simulink library "AnnSteeringBtc"  (R2022b)
settings: Solver=VariableStepAuto  StartTime=0.0  StopTime=10.0  RelTol=1e-3
undefined symbols (not defined in the file or in its folder): frameSize
libraries: dspindex x2, AudioStats x1, FeaturePath x1, HandyTextFile x1, RTC x1
settings Model: Creator=kl13806  LastModifiedBy=kl13806
settings SolverCC: AlgebraicLoopSolver=TrustRegion
settings DebuggingCC: UnconnectedInputMsg=warning  UnconnectedOutputMsg=warning  UnconnectedLineMsg=warning  SFMachineParentedDataDiag=warning
settings ModelReferenceCC: EnableRefExpFcnMdlSchedulingChecks=on
settings RTWCC: DLArmComputeVersion=19.05

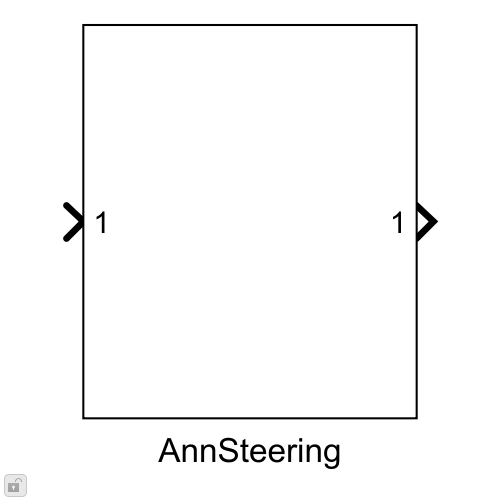
[thumbnail: Simulink's stored preview of the top-level diagram]
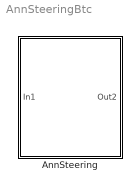
== system AnnSteeringBtc ==
  AnnSteering : Subsystem  mask(Blocklib AnnSteering){Config=[], FeatureName=Steering}
      mask prompts: Config "AnnSteeringConfig"; FeatureName "Feature path name:"
      mask init:
      | blkh=gcbh;
      | Config=BTConfig.Assert(blkh,Config);
      | %Min value to ramp up from
      | minValue = 10^(Config.MinGainDb/20);
      | Config.Validate();
      | BTConfig.InitSetFeatureIfPresent(blkh,'FeatureName');
      mask Callback Config: BTConfig.CallbackHideIfPresent(gcbh,{'FeatureName'});
      mask TypeOptions FeatureName: FeaturePath/FeatureName

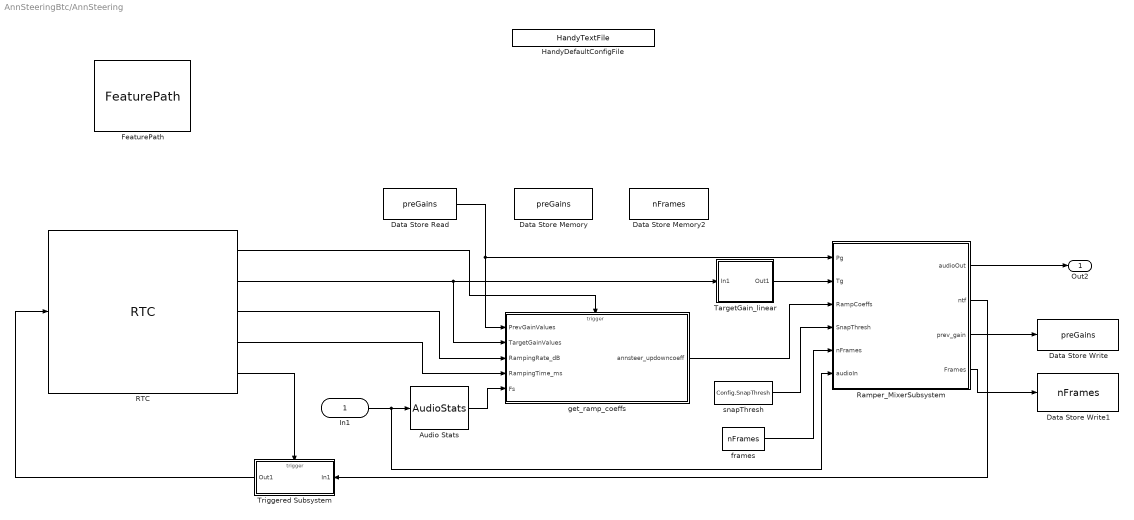
== system AnnSteeringBtc/AnnSteering ==
  In1 : Inport
  Audio Stats : AudioStats/AudioStats  DoSampleRate=on  TypeSampleRate=Inherit: auto  DoCallRate=off  TypeCallRate=Inherit: auto  DoFrameSize=off  TypeFrameSize=Inherit: auto  DoChannelCount=off  TypeChannelCount=Inherit: auto  DoTaskRateFactor=off  TypeTaskRateFactor=Inherit: auto  MacroNameRoot=AUDIO  MacroNameRootEval='AUDIO'  IsMacroNameEval=off  MacroSampleRate=off  MacroCallRate=off  MacroFrameSize=off  MacroChannelCount=off  MacroTaskRateFactor=off  MacroTaskId=off  ValidateSampleRate=off  ValueSampleRate=[]  ValidateCallRate=off  ValueCallRate=[]  ValidateFrameSize=off  ValueFrameSize=[]  ValidateChannelCount=off  ValueChannelCount=[]  ValidateTaskRateFactor=off  ValueTaskRateFactor=[]
  Data Store Memory : DataStoreMemory  DataStoreName=preGains  WriteAfterWriteMsg=warning  InitialValue=Config.Prevgainvalues  ShowAdditionalParam=off  OutDataTypeStr=single
  Data Store Memory2 : DataStoreMemory  DataStoreName=nFrames  InitialValue=zeros(Config.NumAnnOut,Config.NumAnnIn)  ShowAdditionalParam=off  OutDataTypeStr=single
  Data Store Read : DataStoreRead  DataStoreName=preGains  IndexOptions=Index vector (dialog)  Indices=1  OutputSizes=1
  Data Store Write : DataStoreWrite  DataStoreName=preGains  IndexOptions=Index vector (dialog)  Indices=1  OutputSizes=1
  Data Store Write1 : DataStoreWrite  DataStoreName=nFrames  IndexOptions=Index vector (dialog)  Indices=1  OutputSizes=1
  FeaturePath : FeaturePath/FeaturePath  FeatureName=Steering  IsGroup=off  GroupNumber=-1  IsModule=off  TriggerInit=[-245 19 -120 111]
  HandyDefaultConfigFile : HandyTextFile/HandyTextFile  TemplateSource=Config  FileSuffix=Init  OpenDialogOnLoad=off  UseThisBlockName=off  TheDefaultText=|  ShowInLibBrowser=on
      | % $(FILENAME) Setup model parameters for each "Init" callback (e.g. update diagram)
      | sample_rate_in_hertz = 44100;
      | frame_size = 32;
      | sysin_channel_count = 2;
  RTC : RTC/RTC  REQ_Priority=RTC_Mask.NormalPriority  RequestAtInit=off  EnableRequest=on  REQElemName1=target_gain_rtc  REQElemType1=single  REQElemWidth1=length(Config.InitialTargetGainRtc)  REQElemInitial1=Config.InitialTargetGainRtc  REQElemName2=annsteer_rampingRate_rtc  REQElemType2=uint32  REQElemWidth2=length(Config.InitialRampingRateRtc)  REQElemInitial2=Config.InitialRampingRateRtc  REQElemName3=annsteer_rampingTime_rtc  REQElemType3=uint32  REQElemWidth3=length(Config.InitialRampingTimeRtc)  REQElemInitial3=Config.InitialRampingTimeRtc  REQElemType4=uint32  REQElemWidth4=1  REQElemInitial4=[]  REQElemType5=uint32  REQElemWidth5=1  REQElemInitial5=[]  REQElemType6=uint32  REQElemWidth6=1  REQElemInitial6=[]  REQElemType7=uint32  REQElemWidth7=1  REQElemInitial7=[]  REQElemType8=uint32  REQElemWidth8=1  REQElemInitial8=[]  REQElemType9=uint32  REQElemWidth9=1  REQElemInitial9=[]  REQElemType10=uint32  REQElemWidth10=1  REQElemInitial10=[]  EnableResponse=on  EnableRSP_StatusIn=off  RSPElemType1=uint32  RSPElemWidth1=1  RSPElemType2=uint32  RSPElemWidth2=1  RSPElemType3=uint32  RSPElemWidth3=1  RSPElemType4=uint32  RSPElemWidth4=1  RSPElemType5=uint32  RSPElemWidth5=1  RSPElemType6=uint32  RSPElemWidth6=1  RSPElemType7=uint32  RSPElemWidth7=1  RSPElemType8=uint32  RSPElemWidth8=1  RSPElemType9=uint32  RSPElemWidth9=1  RSPElemType10=uint32  RSPElemWidth10=1  EnableNotification=on  EnableNTF_PrepTrig=off  NTFElemType1=uint32  NTFElemWidth1=1  NTFElemType2=uint32  NTFElemWidth2=1  NTFElemType3=uint32  NTFElemWidth3=1  NTFElemType4=uint32  NTFElemWidth4=1  NTFElemType5=uint32  NTFElemWidth5=1  NTFElemType6=uint32  NTFElemWidth6=1  NTFElemType7=uint32  NTFElemWidth7=1  NTFElemType8=uint32  NTFElemWidth8=1  NTFElemType9=uint32  NTFElemWidth9=1  NTFElemType10=uint32  NTFElemWidth10=1  MaskMessageName=Set
  Ramper_MixerSubsystem : Subsystem  TreatAsAtomicUnit=on
  TargetGain_linear : Subsystem
  Triggered Subsystem : Subsystem  TreatAsAtomicUnit=on
  frames : DataStoreRead  DataStoreName=nFrames  IndexOptions=Index vector (dialog)  Indices=1  OutputSizes=1
  get_ramp_coeffs : MATLAB Function  TreatAsAtomicUnit=on
  snapThresh : Constant  Value=Config.SnapThresh  VectorParams1D=off  OutDataTypeStr=single
  Out2 : Outport  VectorParamsAs1DForOutWhenUnconnected=off
  wires:
  RTC/2 -> TargetGain_linear/1(In1), get_ramp_coeffs/2(TargetGainValues)
  Ramper_MixerSubsystem/1(audioOut) -> Out2/1
  Data Store Read/1 -> get_ramp_coeffs/1(PrevGainValues), Ramper_MixerSubsystem/1(Pg)
  RTC/3 -> get_ramp_coeffs/3(RampingRate_dB)
  snapThresh/1 -> Ramper_MixerSubsystem/4(SnapThresh)
  In1/1 -> Ramper_MixerSubsystem/6(audioIn), Audio Stats/1
  Ramper_MixerSubsystem/2(ntf) -> Triggered Subsystem/1(In1)
  RTC/5 -> Triggered Subsystem/Trigger
  Triggered Subsystem/1(Out1) -> RTC/1
  get_ramp_coeffs/1(annsteer_updowncoeff) -> Ramper_MixerSubsystem/3(RampCoeffs)
  Audio Stats/1 -> get_ramp_coeffs/5(Fs)
  Ramper_MixerSubsystem/3(prev_gain) -> Data Store Write/1
  RTC/4 -> get_ramp_coeffs/4(RampingTime_ms)
  RTC/1 -> get_ramp_coeffs/Trigger
  TargetGain_linear/1(Out1) -> Ramper_MixerSubsystem/2(Tg)
  frames/1 -> Ramper_MixerSubsystem/5(nFrames)
  Ramper_MixerSubsystem/4(Frames) -> Data Store Write1/1

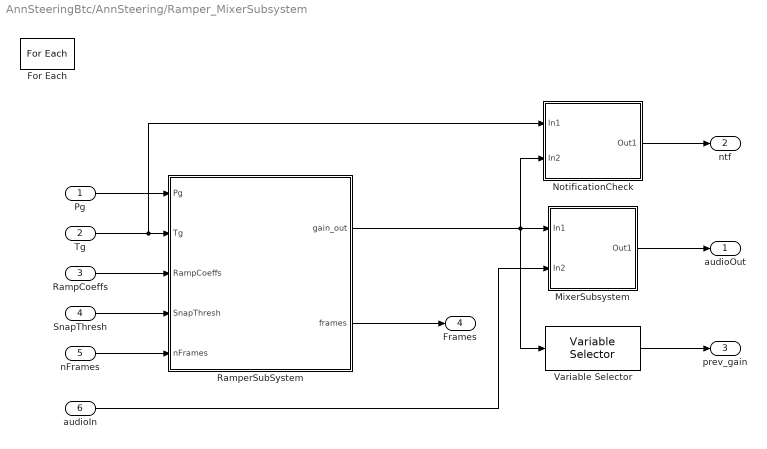
== system AnnSteeringBtc/AnnSteering/Ramper_MixerSubsystem ==
  Pg : Inport  Partition=on  PartitionDimension=1  PartitionWidth=1  PartitionOffset=0
  Tg : Inport  Port=2  Partition=on  PartitionDimension=1  PartitionWidth=1  PartitionOffset=0
  RampCoeffs : Inport  Port=3  Partition=on  PartitionDimension=1  PartitionWidth=1  PartitionOffset=0
  SnapThresh : Inport  Port=4  Partition=on  PartitionDimension=1  PartitionWidth=1  PartitionOffset=0
  nFrames : Inport  Port=5  Partition=on  PartitionDimension=1  PartitionWidth=1  PartitionOffset=0
  audioIn : Inport  Port=6
  For Each : ForEach  DisableCoverage=on
  MixerSubsystem : Subsystem
  NotificationCheck : Subsystem
  RamperSubSystem : Subsystem  TreatAsAtomicUnit=on
  Variable Selector : dspindex/Variable Selector  NumInputs=1  rowsOrCols=Rows  IdxMode=Fixed  Elements=Config.FrameSize  ZerOneIdxMode=One-based  errmode=Clip Index  FillMode=on  FillValues=0
  audioOut : Outport  ConcatenationDimension=2  VectorParamsAs1DForOutWhenUnconnected=off
  ntf : Outport  Port=2  ConcatenationDimension=2  VectorParamsAs1DForOutWhenUnconnected=off
  prev_gain : Outport  Port=3  ConcatenationDimension=1  VectorParamsAs1DForOutWhenUnconnected=off
  Frames : Outport  Port=4  ConcatenationDimension=1  VectorParamsAs1DForOutWhenUnconnected=off
  wires:
  RampCoeffs/1 -> RamperSubSystem/3(RampCoeffs)
  Tg/1 -> RamperSubSystem/2(Tg), NotificationCheck/1(In1)
  Pg/1 -> RamperSubSystem/1(Pg)
  SnapThresh/1 -> RamperSubSystem/4(SnapThresh)
  RamperSubSystem/1(gain_out) -> Variable Selector/1, MixerSubsystem/1(In1), NotificationCheck/2(In2)
  audioIn/1 -> MixerSubsystem/2(In2)
  MixerSubsystem/1(Out1) -> audioOut/1
  NotificationCheck/1(Out1) -> ntf/1
  Variable Selector/1 -> prev_gain/1
  nFrames/1 -> RamperSubSystem/5(nFrames)
  RamperSubSystem/2(frames) -> Frames/1

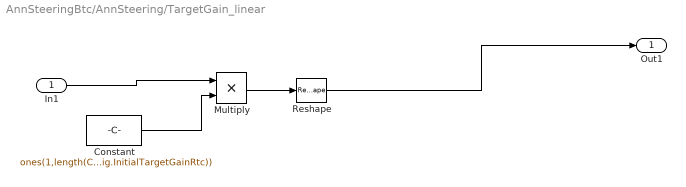
== system AnnSteeringBtc/AnnSteering/TargetGain_linear ==
  In1 : Inport  OutDataTypeStr=single
  Constant : Constant  Value=ones(1,length(Config.InitialTargetGainRtc))  VectorParams1D=off  OutDataTypeStr=single  SampleTime=Inf
  Multiply : Product
  Reshape : Reshape  OutputDimensionality=Customize  OutputDimensions=[Config.NumAnnOut,Config.NumAnnIn]
  Out1 : Outport  VectorParamsAs1DForOutWhenUnconnected=off
  wires:
  Constant/1 -> Multiply/2
  Multiply/1 -> Reshape/1
  In1/1 -> Multiply/1
  Reshape/1 -> Out1/1

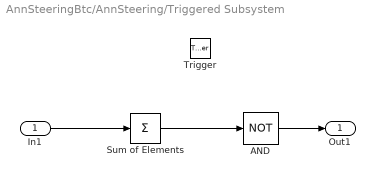
== system AnnSteeringBtc/AnnSteering/Triggered Subsystem ==
  In1 : Inport
  Trigger : TriggerPort  TriggerType=function-call  VariantControl=Variant
  AND : Logic  Operator=NOT  IconShape=distinctive  AllPortsSameDT=off  OutDataTypeStr=boolean
  Sum of Elements : Sum  Inputs=+  CollapseMode=Specified dimension  CollapseDim=2
  Out1 : Outport  VectorParamsAs1DForOutWhenUnconnected=off
  wires:
  In1/1 -> Sum of Elements/1
  Sum of Elements/1 -> AND/1
  AND/1 -> Out1/1

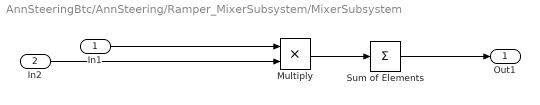
== system AnnSteeringBtc/AnnSteering/Ramper_MixerSubsystem/MixerSubsystem ==
  In1 : Inport
  In2 : Inport  Port=2
  Multiply : Product
  Sum of Elements : Sum  Inputs=+  CollapseMode=Specified dimension  CollapseDim=2
  Out1 : Outport  VectorParamsAs1DForOutWhenUnconnected=off
  wires:
  In2/1 -> Multiply/2
  Multiply/1 -> Sum of Elements/1
  In1/1 -> Multiply/1
  Sum of Elements/1 -> Out1/1

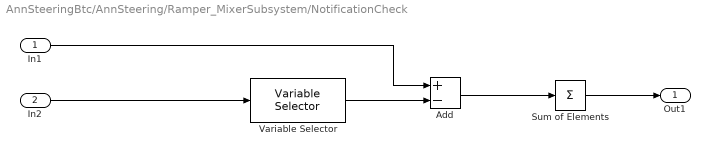
== system AnnSteeringBtc/AnnSteering/Ramper_MixerSubsystem/NotificationCheck ==
  In1 : Inport
  In2 : Inport  Port=2
  Add : Sum  Inputs=+-
  Sum of Elements : Sum  Inputs=+  CollapseMode=Specified dimension  CollapseDim=2
  Variable Selector : dspindex/Variable Selector  NumInputs=1  rowsOrCols=Rows  IdxMode=Fixed  Elements=Config.FrameSize  ZerOneIdxMode=One-based  errmode=Clip Index  FillMode=on  FillValues=0
  Out1 : Outport  VectorParamsAs1DForOutWhenUnconnected=off
  wires:
  Variable Selector/1 -> Add/2
  In1/1 -> Add/1
  In2/1 -> Variable Selector/1
  Sum of Elements/1 -> Out1/1
  Add/1 -> Sum of Elements/1

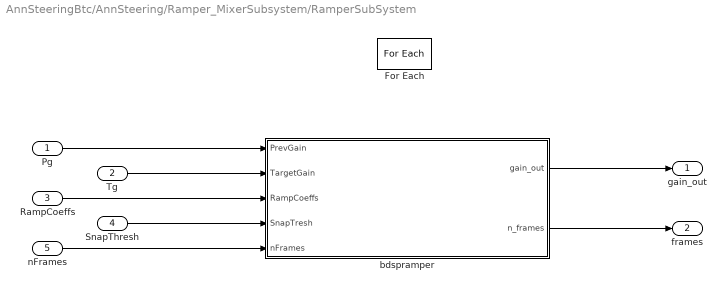
== system AnnSteeringBtc/AnnSteering/Ramper_MixerSubsystem/RamperSubSystem ==
  Pg : Inport  Partition=on  PartitionDimension=2  PartitionWidth=1  PartitionOffset=0
  Tg : Inport  Port=2  Partition=on  PartitionDimension=2  PartitionWidth=1  PartitionOffset=0
  RampCoeffs : Inport  Port=3  Partition=on  PartitionDimension=2  PartitionWidth=1  PartitionOffset=0
  SnapThresh : Inport  Port=4  Partition=on  PartitionDimension=2  PartitionWidth=1  PartitionOffset=0
  nFrames : Inport  Port=5  Partition=on  PartitionDimension=2  PartitionWidth=1  PartitionOffset=0
  For Each : ForEach  DisableCoverage=on
  bdspramper : Subsystem
  gain_out : Outport  ConcatenationDimension=2  VectorParamsAs1DForOutWhenUnconnected=off
  frames : Outport  Port=2  ConcatenationDimension=2  VectorParamsAs1DForOutWhenUnconnected=off
  wires:
  Tg/1 -> bdspramper/2(TargetGain)
  bdspramper/1(gain_out) -> gain_out/1
  RampCoeffs/1 -> bdspramper/3(RampCoeffs)
  Pg/1 -> bdspramper/1(PrevGain)
  SnapThresh/1 -> bdspramper/4(SnapTresh)
  nFrames/1 -> bdspramper/5(nFrames)
  bdspramper/2(n_frames) -> frames/1

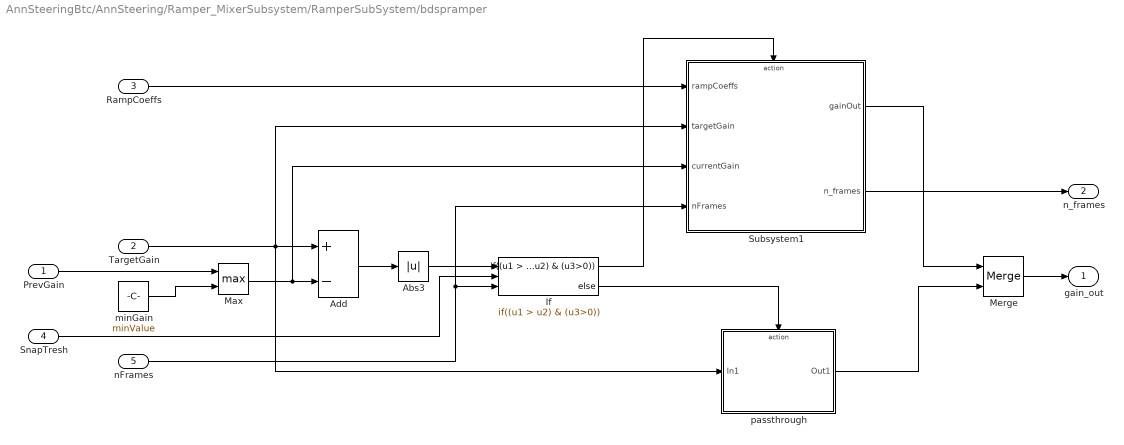
== system AnnSteeringBtc/AnnSteering/Ramper_MixerSubsystem/RamperSubSystem/bdspramper ==
  PrevGain : Inport
  TargetGain : Inport  Port=2
  RampCoeffs : Inport  Port=3
  SnapTresh : Inport  Port=4
  nFrames : Inport  Port=5
  Abs3 : Abs  SaturateOnIntegerOverflow=off
  Add : Sum  Inputs=+-
  If : If  NumInputs=3  IfExpression=(u1 > u2) & (u3>0)
  Max : MinMax  Function=max  Inputs=2
  Merge : Merge
  Subsystem1 : Subsystem
  minGain : Constant  Value=minValue  OutDataTypeStr=single
  passthrough : Subsystem
  gain_out : Outport  VectorParamsAs1DForOutWhenUnconnected=off
  n_frames : Outport  Port=2
  wires:
  Max/1 -> Subsystem1/3(currentGain), Add/2
  passthrough/1(Out1) -> Merge/2
  Merge/1 -> gain_out/1
  Add/1 -> Abs3/1
  TargetGain/1 -> Subsystem1/2(targetGain), passthrough/1(In1), Add/1
  SnapTresh/1 -> If/2
  Abs3/1 -> If/1
  minGain/1 -> Max/2
  PrevGain/1 -> Max/1
  RampCoeffs/1 -> Subsystem1/1(rampCoeffs)
  Subsystem1/1(gainOut) -> Merge/1
  If/1 -> Subsystem1/Action
  If/2 -> passthrough/Action
  nFrames/1 -> If/3, Subsystem1/4(nFrames)
  Subsystem1/2(n_frames) -> n_frames/1

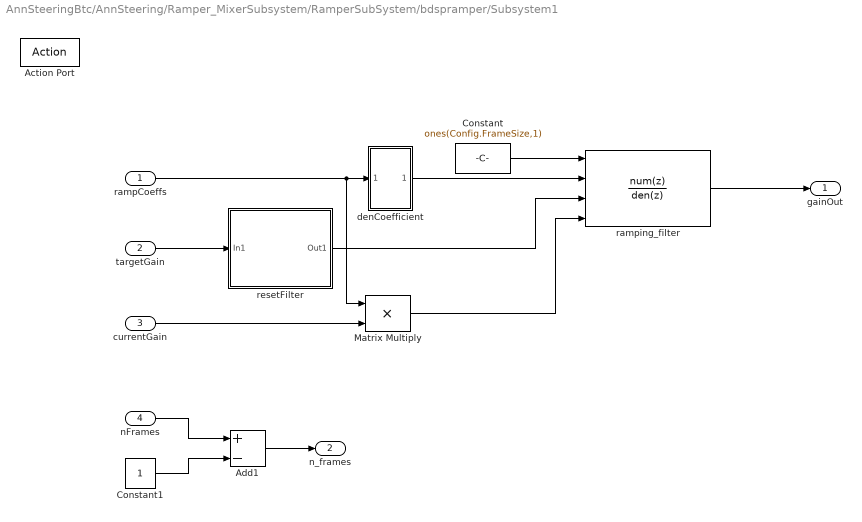
== system AnnSteeringBtc/AnnSteering/Ramper_MixerSubsystem/RamperSubSystem/bdspramper/Subsystem1 ==
  rampCoeffs : Inport
  targetGain : Inport  Port=2
  currentGain : Inport  Port=3
  nFrames : Inport  Port=4
  Action Port : ActionPort
  Add1 : Sum  Inputs=+-
  Constant : Constant  Value=ones(Config.FrameSize,1)  VectorParams1D=off  OutDataTypeStr=single
  Constant1 : Constant  OutDataTypeStr=single
  Matrix Multiply : Product
  denCoefficient : Subsystem
  ramping_filter : DiscreteFilter  Numerator=0  DenominatorSource=Input port  Denominator=[1 -1.0003]  InitialStatesSource=Input port  InitialStates=1.0003  InputProcessing=Columns as channels (frame based)  ExternalReset=Level hold  FilterStructure=Direct form II transposed  a0EqualsOne=on
      settings: InputPortMap=u0,p3,r7,p5
  resetFilter : Subsystem
  gainOut : Outport
  n_frames : Outport  Port=2
  wires:
  Add1/1 -> n_frames/1
  currentGain/1 -> Matrix Multiply/2
  denCoefficient/1(Out1) -> ramping_filter/2
  Constant/1 -> ramping_filter/1
  resetFilter/1(Out1) -> ramping_filter/3
  targetGain/1 -> resetFilter/1(In1)
  rampCoeffs/1 -> denCoefficient/1(In1), Matrix Multiply/1
  ramping_filter/1 -> gainOut/1
  Matrix Multiply/1 -> ramping_filter/4
  nFrames/1 -> Add1/1
  Constant1/1 -> Add1/2

== system AnnSteeringBtc/AnnSteering/Ramper_MixerSubsystem/RamperSubSystem/bdspramper/passthrough ==
  In1 : Inport
  Action Port : ActionPort
  Constant : Constant  Value=ones(Config.FrameSize,1)  VectorParams1D=off  OutDataTypeStr=single
  Multiply : Product
  Out1 : Outport  VectorParamsAs1DForOutWhenUnconnected=off
  wires:
  Multiply/1 -> Out1/1
  Constant/1 -> Multiply/1
  In1/1 -> Multiply/2

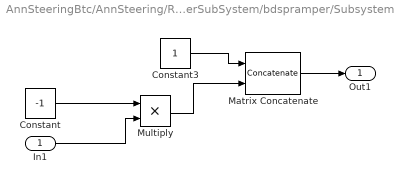
== system AnnSteeringBtc/AnnSteering/Ramper_MixerSubsystem/RamperSubSystem/bdspramper/Subsystem1/denCoefficient ==
  In1 : Inport
  Constant : Constant  Value=-1  OutDataTypeStr=single
  Constant3 : Constant  OutDataTypeStr=single
  Matrix Concatenate : Concatenate  Mode=Multidimensional array  ConcatenateDimension=2
  Multiply : Product
  Out1 : Outport  VectorParamsAs1DForOutWhenUnconnected=off
  wires:
  Constant3/1 -> Matrix Concatenate/1
  Matrix Concatenate/1 -> Out1/1
  Constant/1 -> Multiply/1
  Multiply/1 -> Matrix Concatenate/2
  In1/1 -> Multiply/2

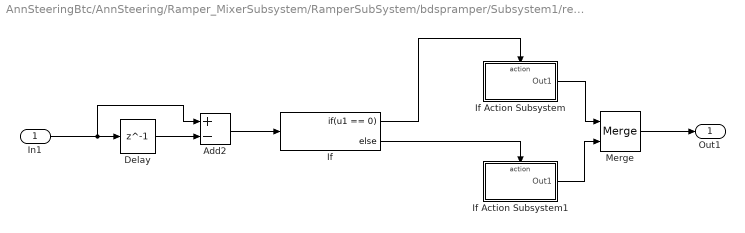
== system AnnSteeringBtc/AnnSteering/Ramper_MixerSubsystem/RamperSubSystem/bdspramper/Subsystem1/resetFilter ==
  In1 : Inport
  Add2 : Sum  Inputs=+-
  Delay : Delay  DelayLength=1
  If : If  IfExpression=u1 == 0
  If Action Subsystem : Subsystem  TreatAsAtomicUnit=on
  If Action Subsystem1 : Subsystem  TreatAsAtomicUnit=on
  Merge : Merge
  Out1 : Outport  VectorParamsAs1DForOutWhenUnconnected=off
  wires:
  Add2/1 -> If/1
  Delay/1 -> Add2/2
  In1/1 -> Add2/1, Delay/1
  If/1 -> If Action Subsystem/Action
  If/2 -> If Action Subsystem1/Action
  If Action Subsystem/1(Out1) -> Merge/1
  If Action Subsystem1/1(Out1) -> Merge/2
  Merge/1 -> Out1/1

== system AnnSteeringBtc/AnnSteering/Ramper_MixerSubsystem/RamperSubSystem/bdspramper/Subsystem1/resetFilter/If Action Subsystem ==
  Action Port : ActionPort
  Constant : Constant  Value=0  OutDataTypeStr=boolean
  Out1 : Outport  VectorParamsAs1DForOutWhenUnconnected=off
  wires:
  Constant/1 -> Out1/1

== system AnnSteeringBtc/AnnSteering/Ramper_MixerSubsystem/RamperSubSystem/bdspramper/Subsystem1/resetFilter/If Action Subsystem1 ==
  Action Port : ActionPort
  Constant : Constant  OutDataTypeStr=boolean
  Out1 : Outport  VectorParamsAs1DForOutWhenUnconnected=off
  wires:
  Constant/1 -> Out1/1

== matlab function AnnSteeringBtc/AnnSteering/get_ramp_coeffs ==
  data: PrevGainValues input; TargetGainValues input; annsteer_updowncoeff output; RampingRate_dB input; RampingTime_ms input; Fs input; minValue parameter; nFrames data_store_memory; frameSize parameter
  events: trigger input FUNCTION_CALL_EVENT
function annsteer_updowncoeff = fcn(PrevGainValues, TargetGainValues,RampingRate_dB,RampingTime_ms, Fs, minValue, frameSize)

global nFrames

[numAnnOut,numAnnInp] = size(PrevGainValues);
TargetGain = reshape(TargetGainValues,numAnnOut,numAnnInp);
RampingRate = single(reshape(RampingRate_dB,numAnnOut,numAnnInp));
RampingTime = single(reshape(RampingTime_ms,numAnnOut,numAnnInp));

% Nudge the gain values a bit if they are sitting at zero.
% If current gain is zero, replace with a value very close to zero. What we
% really want is a value which is on the edge of perception - not too small
% or large. If the value is too small, we'll waste some of our ramp time
% in perceived silence. If the value is too large, the audio will lurch
% into perceptability at the start of the ramp.
PrevGain = max(PrevGainValues, minValue);
TargetGain  = max(TargetGain, minValue);

% In order to have the desired ramp time, the slope must vary dependent
% on the gain difference between target and current value.
% Equivalent ramp rate is therefore calculated as follows:
GainFactor_dB = abs(20.*log10(TargetGain./PrevGain));   
if (~RampingRate_dB)     
    RampingRate = (GainFactor_dB.*1000)./RampingTime;
end

quantum_ms = 1000 * frameSize / Fs;
nFrames = ceil(((GainFactor_dB.*1000)./RampingRate) ./ quantum_ms);
quantized_rampTime_ms = nFrames .* quantum_ms;
RampingRate = (GainFactor_dB.*1000)./quantized_rampTime_ms;

GainDiff = TargetGain-PrevGain;
% Conver db/s to ramping filter coeffs
annsteer_updowncoeff = single(zeros(numAnnOut,numAnnInp));
annsteer_updowncoeff(GainDiff>=0)  = 10.^((single(RampingRate(GainDiff>=0))./Fs)./20);
annsteer_updowncoeff(GainDiff<0)  = 10.^((-single(RampingRate(GainDiff<0))./Fs)./20);
